simulink model "RocketAirBrake_Simulation_Alan"  (R2018b)
settings: Solver=FixedStepAuto  StartTime=0.0  StopTime=30  FixedStep=0.001  RelTol=1e-3
libraries: embdlinuxlib x6
(part 1 of 3)
settings Model: Creator=benkl  LastModifiedBy=Alan
settings SolverCC: AlgebraicLoopSolver=LineSearch

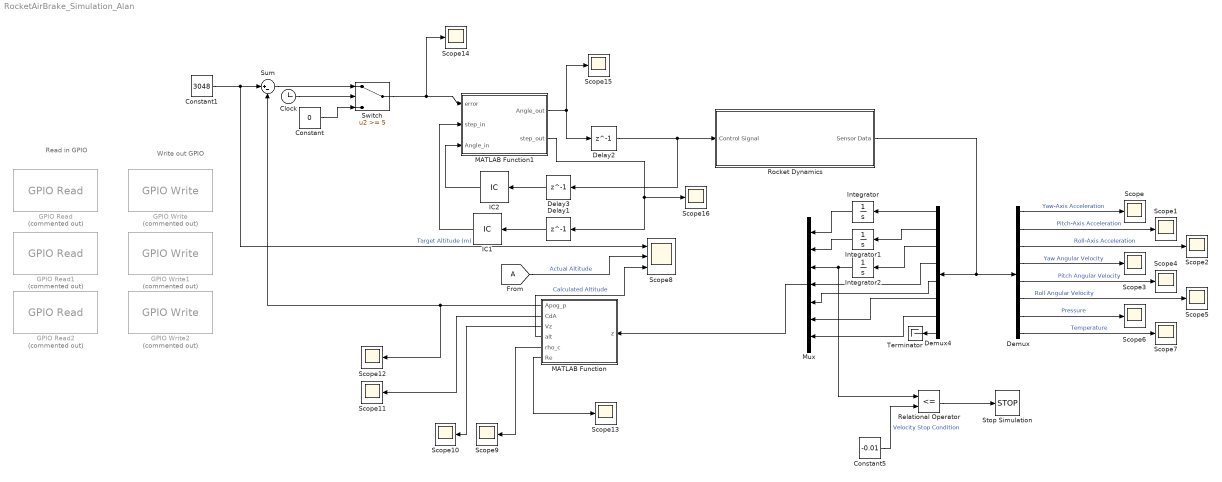
== system RocketAirBrake_Simulation_Alan ==
  note: Read in GPIO
  note: Write out GPIO
  Clock : Clock
  Constant : Constant  Value=0
  Constant1 : Constant  Value=3048
  Constant5 : Constant  Value=-0.01
  Delay1 : Delay  DelayLength=1  InitialCondition=0
  Delay2 : Delay  DelayLength=1  InitialCondition=0
  Delay3 : Delay  DelayLength=1  InitialCondition=0
  Demux : Demux  Outputs=8
  Demux4 : Demux  Outputs=8
  GPIO Read : embdlinuxlib/GPIO Read  Commented=on  board=Model B+  gpio=4  internalResistor=Off  sampleTime=0.1  direction=Input  blockPlatform=Raspberry Pi
      settings: SourceProductName=Simulink Support Package for Raspberry Pi Hardware  SourceProductBaseCode=RASPPI
  GPIO Read1 : embdlinuxlib/GPIO Read  Commented=on  board=Model B+  gpio=4  internalResistor=Off  sampleTime=0.1  direction=Input  blockPlatform=Raspberry Pi
      settings: SourceProductName=Simulink Support Package for Raspberry Pi Hardware  SourceProductBaseCode=RASPPI
  GPIO Read2 : embdlinuxlib/GPIO Read  Commented=on  board=Model B+  gpio=4  internalResistor=Off  sampleTime=0.1  direction=Input  blockPlatform=Raspberry Pi
      settings: SourceProductName=Simulink Support Package for Raspberry Pi Hardware  SourceProductBaseCode=RASPPI
  GPIO Write : embdlinuxlib/GPIO Write  Commented=on  board=Model B+  gpio=17  direction=Output  blockPlatform=Raspberry Pi
      settings: SourceProductName=Simulink Support Package for Raspberry Pi Hardware  SourceProductBaseCode=RASPPI
  GPIO Write1 : embdlinuxlib/GPIO Write  Commented=on  board=Model B+  gpio=17  direction=Output  blockPlatform=Raspberry Pi
      settings: SourceProductName=Simulink Support Package for Raspberry Pi Hardware  SourceProductBaseCode=RASPPI
  GPIO Write2 : embdlinuxlib/GPIO Write  Commented=on  board=Model B+  gpio=17  direction=Output  blockPlatform=Raspberry Pi
      settings: SourceProductName=Simulink Support Package for Raspberry Pi Hardware  SourceProductBaseCode=RASPPI
  IC1 : InitialCondition  Value=0
  IC2 : InitialCondition  Value=0
  Integrator : Integrator
  Integrator1 : Integrator
  Integrator2 : Integrator
  MATLAB Function : MATLAB Function  TreatAsAtomicUnit=on
  MATLAB Function1 : MATLAB Function  TreatAsAtomicUnit=on
  Mux : Mux  Inputs=7
  Relational Operator : RelationalOperator  Operator=<=  OutDataTypeStr=boolean  RndMeth=Simplest
  Rocket Dynamics : Subsystem
  Scope{,1..7,9..16} (16 alike) : Scope
  Scope8 : Scope  NumInputPorts=3
  Stop Simulation : Stop
  Sum : Sum  Inputs=|+-
  Switch : Switch  Threshold=5
  Terminator : Terminator
  wires:
  Demux/1 -> Scope/1  "Yaw-Axis Acceleration"
  Demux/2 -> Scope1/1  "Pitch-Axis Acceleration"
  Rocket Dynamics/1(Sensor Data) -> Demux4/1, Demux/1
  Demux/8 -> Scope7/1  "Temperature"
  Demux/3 -> Scope2/1  "Roll-Axis Acceleration"
  Demux/4 -> Scope3/1  "Yaw Angular Velocity"
  Demux/5 -> Scope4/1  "Pitch Angular Velocity"
  Demux/6 -> Scope5/1  "Roll Angular Velocity"
  Demux/7 -> Scope6/1  "Pressure"
  [A] -> Scope8/2  "Actual Altitude"
  Mux/1 -> MATLAB Function/1(z)
  Demux4/2 -> Integrator1/1
  Integrator1/1 -> Mux/2
  Demux4/1 -> Integrator/1
  Integrator/1 -> Mux/1
  Integrator2/1 -> Relational Operator/1, Mux/3
  Demux4/3 -> Integrator2/1
  Demux4/4 -> Mux/4
  Demux4/5 -> Mux/5
  Demux4/6 -> Mux/6
  Demux4/7 -> Mux/7
  Demux4/8 -> Terminator/1
  MATLAB Function/4(alt) -> Scope8/3  "Calculated Altitude"
  MATLAB Function/5(rho_c) -> Scope9/1
  MATLAB Function/1(Apog_p) -> Sum/2, Scope12/1
  MATLAB Function/2(CdA) -> Scope11/1
  MATLAB Function/6(Re) -> Scope13/1
  Constant5/1 -> Relational Operator/2  "Velocity Stop Condition"
  MATLAB Function/3(Vz) -> Scope10/1
  Relational Operator/1 -> Stop Simulation/1
  Constant1/1 -> Scope8/1, Sum/1  "Target Altitude (m)"
  Delay1/1 -> IC1/1
  MATLAB Function1/2(step_out) -> Delay1/1, Scope16/1
  IC1/1 -> MATLAB Function1/2(step_in)
  MATLAB Function1/1(Angle_out) -> Delay2/1, Scope15/1
  Delay2/1 -> Delay3/1, Rocket Dynamics/1(Control Signal)
  Sum/1 -> Switch/1
  Switch/1 -> MATLAB Function1/1(error), Scope14/1
  Clock/1 -> Switch/2
  Constant/1 -> Switch/3
  IC2/1 -> MATLAB Function1/3(Angle_in)
  Delay3/1 -> IC2/1

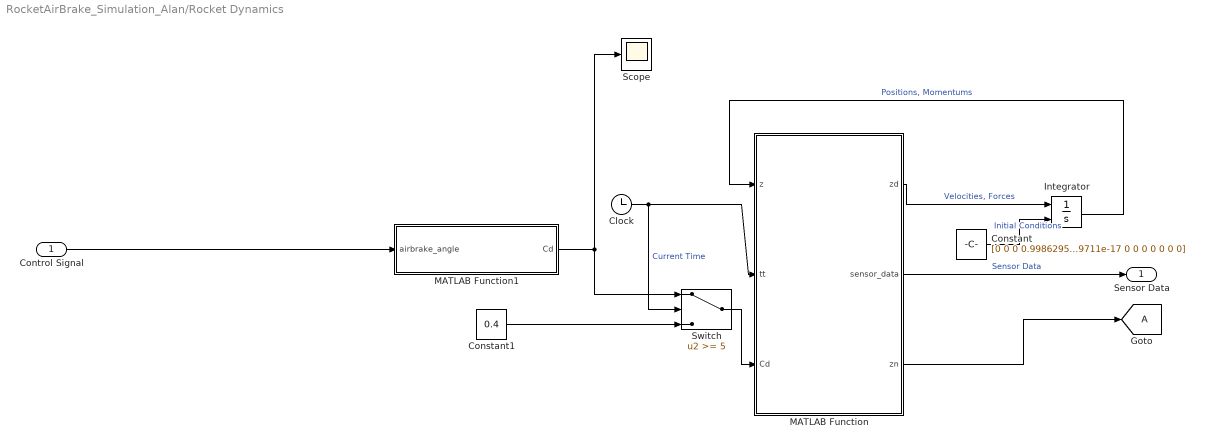
== system RocketAirBrake_Simulation_Alan/Rocket Dynamics ==
  Control Signal : Inport
  Clock : Clock
  Constant : Constant  Value="[0\t0\t0\t0.998629534754574\t-0.0523359562429438\t1.92279183879711e-17\t0\t0\t0\t0\t0\t0\t0]"
  Constant1 : Constant  Value=0.4
  Integrator : Integrator  InitialConditionSource=external
  MATLAB Function : MATLAB Function  TreatAsAtomicUnit=on
  MATLAB Function1 : MATLAB Function  TreatAsAtomicUnit=on
  Scope : Scope
  Switch : Switch  Threshold=5
  Sensor Data : Outport
  tag scope: A=global
  wires:
  Clock/1 -> MATLAB Function/2(tt), Switch/2  "Current Time"
  Integrator/1 -> MATLAB Function/1(z)  "Positions, Momentums"
  MATLAB Function/1(zd) -> Integrator/1  "Velocities, Forces"
  Constant/1 -> Integrator/2  "Initial Conditions"
  MATLAB Function/2(sensor_data) -> Sensor Data/1  "Sensor Data"
  Control Signal/1 -> MATLAB Function1/1(airbrake_angle)
  MATLAB Function/3(zn) -> [A]
  Switch/1 -> MATLAB Function/3(Cd)
  Constant1/1 -> Switch/3
  MATLAB Function1/1(Cd) -> Switch/1, Scope/1

== matlab function RocketAirBrake_Simulation_Alan/MATLAB Function ==
  data: z input; Apog_p output; CdA output; Vz output; alt output; rho_c output; Re output
function [Apog_p,CdA,Vz,alt,rho_c,Re] = feedback(z)

% Vx = z(1);
% Vy = z(2);
% Vz = z(3);
% psi_dot = z(4);
% theta_dot = z(5);
% phi_dot = z(6);
Pr = z(7);

g = 9.81;
% Ix = 2.1638;
% Iy = 2.1638;
% Iz = 0.0016;
m = 15.7210;
Ar=0.010751315458748; % Rocket aerodynamic reference area
L = -0.0065;
To = 287;
Po = 85000;
Rconst = 287.058;
epsilon = 15;
u = 1.6*(10^-5);
c = 2;

T = To*((Pr/Po)^(L*Rconst/g));
rho_c = Pr/(Rconst*T);
alt = -(Rconst*T/g)*log(Pr/Po);
Vz = z(3);
Re = abs(Vz*c/u);
Cd = 2*sind(epsilon)*sind(epsilon) + 1/sqrt(Re);
Apog_p = alt + m/(Cd*Ar*rho_c)*log((Cd*Ar*rho_c*Vz*Vz/(2*m*g))+1);
CdA = Cd*Ar;
